simulink model "rtwdemo_targetsettings"  (Simulink 7.6)
settings: Solver=FixedStepDiscrete  StartTime=0.0  StopTime=1  FixedStep=1  RelTol=1e-3
libraries: rtwdemowidgets x2
Description:
  | Specifying Target Environment Settings
settings Model: Creator=The MathWorks Inc.  ExtModeTrigMode=oneshot  ExtModeArmWhenConnect=off  ExtModeAutoUpdateStatusClock=off
settings MATStruct: SampleTime=1  Offset=0  Priority=[20.0]
settings DataIOCC: LimitDataPoints=off  SaveOutput=off  SaveTime=off  SignalLoggingName=logsOut
settings OptimizationCC: InlineParams=on  InlineInvariantSignals=on  StateBitsets=on  DataBitsets=on  UseTempVars=on  EfficientFloat2IntCast=on  EfficientMapNaN2IntZero=off
settings DebuggingCC: CheckExecutionContextPreStartOutputMsg=on  CheckExecutionContextRuntimeOutputMsg=on  SolverPrmCheckMsg=none  InheritedTsInSrcMsg=none  IntegerOverflowMsg=none  StrictBusMsg=ErrorOnBusTreatedAsVector
settings HardwareCC: ProdIntDivRoundTo=Zero  ProdEndianess=LittleEndian  ProdHWDeviceType=Generic->32-bit Embedded Processor  TargetHWDeviceType=Generic->32-bit Embedded Processor
settings ModelReferenceCC: UpdateModelReferenceTargets=IfOutOfDate
settings RTWCC: GenerateReport=on  RTWVerbose=off  ProcessScript=grt_make_rtw_hook  LaunchReport=on
settings CodeAppCC: ForceParamTrailComments=on
settings GRTTargetCC: TargetFcnLib=ansi_tfl_tmw.mat

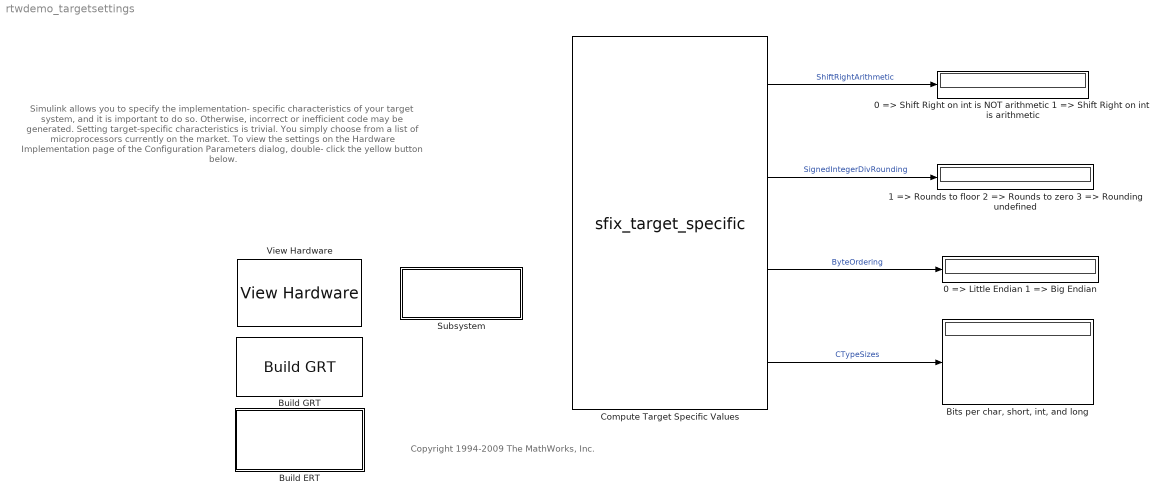
== system rtwdemo_targetsettings ==
  note: Simulink allows you to specify the implementation-
      | specific characteristics of your target system, and
      | it is important to do so.  Otherwise, incorrect or
      | inefficient code may be generated.
      |
      | Setting target-specific characteristics is trivial.
      | You simply choose from a list of microprocessors
      | currently on the market.
      |
      | To view the settings on the Hardware Implementation
      | page of the Configuration Parameters dialog, double-
      | click the yellow button below.
  note: Copyright 1994-2009 The MathWorks, Inc.
  "0 => Little Endian 1 => Big Endian   " : Display
  "0 => Shift Right on int is NOT arithmetic 1 => Shift Right on int is arithmetic    " : Display
  1 => Rounds to floor 2 => Rounds to zero 3 => Rounding undefined : Display
  "Bits per char, short, int, and long" : Display
  Build ERT : Subsystem  mask{attrib_overrides={}}
      mask prompts: attrib_overrides "List of attributes to preserve (cell of strings):"
      mask help: Enter the attributes of the configuration set that you want preserved. Otherwise, the default configuration script will override your current settings.
      settings: OpenFcn=|
      | model=bdroot;
      |                   overrides=get_param(gcb,'attrib_overrides');
      | try
      |   rtwconfiguredemo(model,'noop',false,overrides);
      |   rtwbuilddemomodel(model);
      | catch
      |   error(lasterr);
      | end
      |   clear model overrides;
      mask Display:
      | disp(['Generate Code Using\n',...
      | 	  'Real-Time Workshop\n',...
      | 	  'Embedded Coder\n'...
      | 	  '(double-click)'])
  Build GRT : rtwdemowidgets/Build GRT  SystemSampleTime=-1  attrib_overrides={}
  Compute Target Specific Values : S-Function  FunctionName=sfix_target_specific  EnableBusSupport=off
      mask Type: Fixed-Point Target Specific
      mask Description: Used to get information about a fixed point target compiler/processor.
      mask Help: helpview([docroot '/toolbox/rtw/helptargets.map'], 'rtw_hardware_implementation');
      mask Display:
      | port_label('output',1,'Shift Right on int is arithmetic' );
      | port_label('output',2,'Signed integer division rounding' );
      | port_label('output',3,'Byte ordering' );
      | port_label('output',4,'Bits per char, short, int, long' );
  Subsystem : Subsystem
      mask Display: disp(['My microprocessor\nis not listed ..','.        '])
  View Hardware : rtwdemowidgets/View Hardware  SystemSampleTime=-1
  wires:
  Compute Target Specific Values/3 -> "0 => Little Endian 1 => Big Endian   "/1  "ByteOrdering"
  Compute Target Specific Values/4 -> "Bits per char, short, int, and long"/1  "CTypeSizes"
  Compute Target Specific Values/1 -> "0 => Shift Right on int is NOT arithmetic 1 => Shift Right on int is arithmetic    "/1  "ShiftRightArithmetic"
  Compute Target Specific Values/2 -> 1 => Rounds to floor 2 => Rounds to zero 3 => Rounding undefined/1  "SignedIntegerDivRounding"

== system rtwdemo_targetsettings/Build ERT ==

== system rtwdemo_targetsettings/Subsystem ==
  note: If your system is not listed and you are not certain of its values, use the code generated
      | by this model to compute the necessary C compiler and target hardware settings.
      |
      | If you use a cross-development system that includes a source level debugger, first
      | configure the model for your intended target. Then generate code and build an executable
      | using your target development system (for more details about retrieving file and path
      | information, see the documentation on the Real-Time Workshop Build Information API).
      | Download the executable to the target and set breakpoints at the model output code for
      | each of the outports of the model.  Run a debugging session and observe the behavior
      | of the code as it executes on the target. As you step through the code the values for the
      | various characteristics are computed.
      |
      | If your target development system does not support source level debugging, you may have to
      | generate code and add printf statements or other code that enables you to obtain the
      | results.
      |
      | Once you've obtained your target settings, enter them into the Hardware Implementation
      | page via a 'Generic->Custom' device type.
